simulink model "power_pwm"  (Simulink 6.0)
settings: Solver=ode23tb  SolverMode=SingleTasking  StartTime=0.0  StopTime=1  MaxStep=10e-6  RelTol=1e-4
libraries: powerlib x4, powerlib_extras x1
settings Model: Creator=patrice  LastModifiedBy=batserve  ExtModeTrigMode=oneshot  ExtModeArmWhenConnect=off  ExtModeAutoUpdateStatusClock=off
settings DataIOCC: ExternalInput=[]  LimitDataPoints=off  SaveOutput=off  TimeSaveName=t  SignalLoggingName=sigsOut
settings OptimizationCC: BlockReduction=off  BooleanDataType=off
settings DebuggingCC: CheckExecutionContextPreStartOutputMsg=on  CheckExecutionContextRuntimeOutputMsg=on  SolverPrmCheckMsg=none  UnconnectedInputMsg=none  UnconnectedOutputMsg=none
settings HardwareCC: TargetUnknown=on
settings RTWCC: TemplateMakefile=grt_unix.tmf

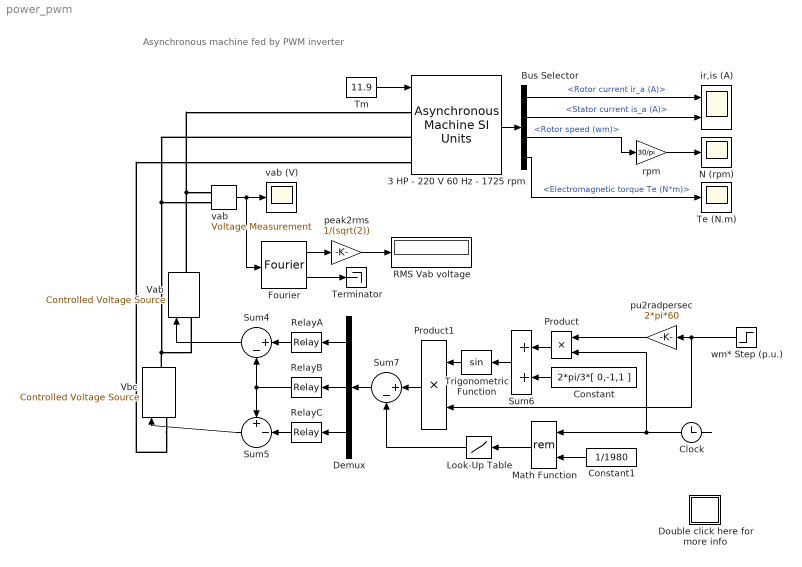
== system power_pwm ==
  note: Asynchronous machine fed by PWM inverter
  3 HP - 220 V 60 Hz - 1725 rpm : powerlib/Machines/Asynchronous Machine SI Units  PresetModel=No  ShowDetailedParameters=on  RotorType=Squirrel-cage  ReferenceFrame=Stationary  NominalParameters=[ 3*746, 220, 60 ]  Stator="[ 0.435  2*2.0e-3 ]"  Rotor="[ 0.816  2.0e-3 ]"  Lm=69.31e-3  Mechanical="[ 0.089  0  2 ]"  InitialConditions="[ 1,0   0,0,0   0,0,0 ]"  Units=1  LoadFlowParameters=0
  Bus Selector : BusSelector  DialogController=Simulink.DDGSource_Bus  OutputSignals=Rotor measurements.Rotor current ir_a (A),Stator measurements.Stator current is_a (A),Mechanical.Rotor speed (wm),Mechanical.Electromagnetic torque Te (N*m)
  Clock : Clock
      settings: Decimation=10
  Constant : Constant  Orientation=left  Value=2*pi/3*[ 0,-1,1 ]
  Constant1 : Constant  Orientation=left  Value=1/1980
  Demux : Demux  Orientation=left  Outputs=3
  Double click here for more info : Subsystem
      mask Display: disp('?')
  Fourier : powerlib_extras/Measurements/Fourier  f1=60  n=1
  Look-Up Table : Lookup  Orientation=left  DialogController=Simulink.DDGSource  InputValues="[0 0.25  0.75  1] / 1980"  OutputValues="[0  1  -1  0]"  SaturateOnIntegerOverflow=on
  Math Function : Math  Orientation=left  Operator=rem  SaturateOnIntegerOverflow=on
  N (rpm) : Scope
      settings: TimeRange=1  YMin=-200  YMax=1800  DataFormat=Structure
  Product : Product  Orientation=left  SaturateOnIntegerOverflow=on  InputSameDT=on
  Product1 : Product  Orientation=left  SaturateOnIntegerOverflow=on  InputSameDT=on
  RMS Vab voltage : Display
      settings: Decimation=100
  RelayA : Relay  Orientation=left  OnSwitchValue=0  OffSwitchValue=0  OnOutputValue=220*sqrt(2/3)  OffOutputValue=-220*sqrt(2/3)
  RelayB : Relay  Orientation=left  OnSwitchValue=0  OffSwitchValue=0  OnOutputValue=220*sqrt(2/3)  OffOutputValue=-220*sqrt(2/3)
  RelayC : Relay  Orientation=left  OnSwitchValue=0  OffSwitchValue=0  OnOutputValue=220*sqrt(2/3)  OffOutputValue=-220*sqrt(2/3)
  Sum4 : Sum  Orientation=left  Inputs=|+-  SaturateOnIntegerOverflow=on  InputSameDT=on
  Sum5 : Sum  Orientation=left  Inputs=+-|  SaturateOnIntegerOverflow=on  InputSameDT=on
  Sum6 : Sum  Orientation=left  SaturateOnIntegerOverflow=on  InputSameDT=on
  Sum7 : Sum  Orientation=left  Inputs=|+-  SaturateOnIntegerOverflow=on  InputSameDT=on
  Te (N.m) : Scope
      settings: YMin=-30  YMax=100  DataFormat=Structure
  Terminator : Terminator
  Tm : Constant  Value=11.9
  Trigonometric Function : Trigonometry  Orientation=left
  Vab : powerlib/Electrical Sources/Controlled Voltage Source  Description=source block  Orientation=up  Initialize=on  Amplitude=0  Phase=0  Frequency=0  Measurements=None
      settings: AttributesFormatString=\n
  Vbc : powerlib/Electrical Sources/Controlled Voltage Source  Description=source block  Orientation=up  Initialize=on  Amplitude=0  Phase=0  Frequency=0  Measurements=None
      settings: AttributesFormatString=\n
  ir,is (A) : Scope  NumInputPorts=2
      settings: YMin=-90~-90  YMax=90~90  DataFormat=Structure
  peak2rms : Gain  Gain=1/(sqrt(2))  SaturateOnIntegerOverflow=on
  pu2radpersec : Gain  Orientation=left  Gain=2*pi*60  SaturateOnIntegerOverflow=on
  rpm : Gain  Gain=30/pi  SaturateOnIntegerOverflow=on
  vab : powerlib/Measurements/Voltage Measurement  Tag=PoWeRsYsTeMmEaSuReMeNt  PhasorSimulation=off  OutputType=Magnitude  PSBequivalent=0
  vab (V) : Scope
      settings: TimeRange=0.1  YMin=-400  YMax=400  DataFormat=Structure
  wm* Step (p.u.) : Step  Orientation=left  Time=0  SampleTime=0
  wires:
  RelayA/1 -> Sum4/1
  RelayC/1 -> Sum5/2
  RelayB/1 -> Sum5/1, Sum4/2
  Demux/2 -> RelayB/1
  Demux/3 -> RelayC/1
  Demux/1 -> RelayA/1
  Sum7/1 -> Demux/1
  pu2radpersec/1 -> Product/1
  Sum6/1 -> Trigonometric Function/1
  Trigonometric Function/1 -> Product1/1
  Product1/1 -> Sum7/1
  wm* Step (p.u.)/1 -> pu2radpersec/1, Product1/2
  Look-Up Table/1 -> Sum7/2
  Clock/1 -> Product/2, Math Function/1
  Math Function/1 -> Look-Up Table/1
  Constant1/1 -> Math Function/2
  Product/1 -> Sum6/1
  Constant/1 -> Sum6/2
  Fourier/1 -> peak2rms/1
  peak2rms/1 -> RMS Vab voltage/1
  Fourier/2 -> Terminator/1
  Bus Selector/4 -> Te (N.m)/1  "<Electromagnetic torque Te (N*m)>"
  rpm/1 -> N (rpm)/1
  Tm/1 -> 3 HP - 220 V 60 Hz - 1725 rpm/1
  Sum4/1 -> Vab/1
  Sum5/1 -> Vbc/1
  vab/1 -> vab (V)/1, Fourier/1
  Bus Selector/1 -> ir,is (A)/1  "<Rotor current ir_a (A)>"
  3 HP - 220 V 60 Hz - 1725 rpm/1 -> Bus Selector/1
  Bus Selector/2 -> ir,is (A)/2  "<Stator current is_a (A)>"
  Bus Selector/3 -> rpm/1  "<Rotor speed (wm)>"
  connections:
  Vbc/LConn1 -- 3 HP - 220 V 60 Hz - 1725 rpm/LConn3
  Vab/RConn1 -- 3 HP - 220 V 60 Hz - 1725 rpm/LConn1 -- vab/LConn1
  3 HP - 220 V 60 Hz - 1725 rpm/LConn2 -- Vbc/RConn1 -- Vab/LConn1 -- vab/LConn2

== system power_pwm/Double click here for more info ==
  note: Demonstration
  note: Circuit Description
  note: This demonstration illustrates use of the asynchronous machine
      | in an open-loop speed control on a 3 HP 220 V industrial motor
  note: A three-phase motor rated 3 HP, 220 V, 1725 rpm is fed by a sinusoidal PWM inverter. The base frequency
      | of the sinusoidal reference wave is 60 Hz while the triangular carrier wave's frequency is set to 1980 Hz.
      | The PWM inverter is built entirely with standard Simulink blocks. Its output goes through Controlled Voltage
      | Source blocks before being applied to the Asynchronous Machine block's stator windings. The machine's
      | rotor is short-circuited. Its stator leakage inductance Lls is set to twice its actual value to simulate the
      | effect of a smoothing reactor placed between the inverter and the machine. The load torque applied to the
      | machine's shaft is constant and set to its nominal value of 11.9 N.m.
      |
      | The motor is started from stall. The speed setpoint is set to 1.0 pu, or 1725 rpm. This speed is reached
      | after 0.9 s.
  note: Take a look at the simulation parameters. The Maximum time step has been limited to 10 microseconds.
      | This is required due to the relatively high switching frequency (1980 Hz) of the inverter.
      |
      | Observe that the rotor and stator currents are quite "noisy," despite the use of a smoothing reactor. The noise
      | introduced by the PWM inverter is also observed in the electromagnetic torque waveform Te. However, the
      | motor's inertia prevents this noise from appearing in the motor's speed waveform.
      |
      | The RMS value of the fundamental component of the line voltage at the machine's stator terminals is extracted
      | with a Fourier block, which can be found in the Measurements group of the Extras library.
      |
      | Finally, observe the PWM inverter's output. Use the zoom on the vab oscilloscope to zoom in on the waveform.
  note: Louis-A. Dessaint and R. Champagne (Ecole de Technologie Superieure, Montreal)
